simulink subsystem "SerialTX"  (R2022a)
settings: Solver=VariableStepAuto  StartTime=0.0  StopTime=10.0  RelTol=1e-3
undefined symbols (not defined in the file): A0, A1, PTB2, PTB3
libraries: frdmk64flib x3
settings Model: Creator=bkfre  LastModifiedBy=bkfre

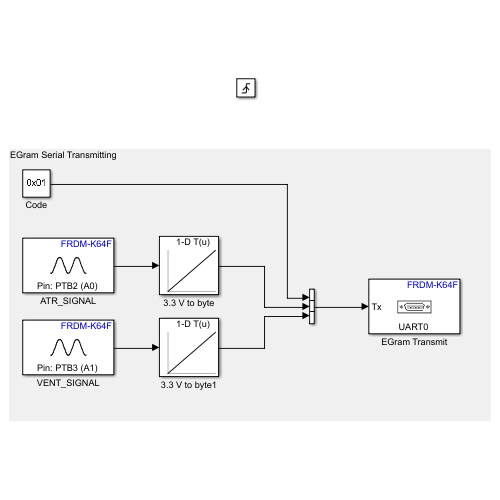
[thumbnail: Simulink's stored preview of the top-level diagram]
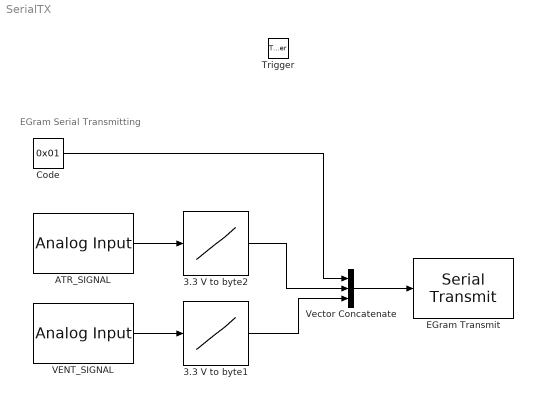
== system SerialTX ==
  note: EGram Serial Transmitting
  Trigger : TriggerPort  VariantControl=(inherit)  PortDimensions=1
  3.3 V to byte1 : Lookup_n-D  NumberOfTableDimensions=1  BreakpointsForDimension1=[0,3.3]  Table=[0,255]  ExtrapMethod=Clip  InternalRulePriority=Speed  OutDataTypeStr=uint8  RndMeth=Simplest
  3.3 V to byte2 : Lookup_n-D  NumberOfTableDimensions=1  BreakpointsForDimension1=[0,3.3]  Table=[0,255]  ExtrapMethod=Clip  InternalRulePriority=Speed  OutDataTypeStr=uint8  RndMeth=Simplest
  ATR_SIGNAL : frdmk64flib/Analog Input  Whichpin=PTB2 (A0)  SampleTime=-1
  Code : Constant  Value=0x01  OutDataTypeStr=uint8
  EGram Transmit : frdmk64flib/Serial Transmit  SCIModule=0  Baudrate=uint32(9600)  Parity=None  StopBits=1  HardwareFlowControl=None  ByteOrder=LittleEndian  BlockingMode=on  OutputStatus=off
  VENT_SIGNAL : frdmk64flib/Analog Input  Whichpin=PTB3 (A1)  SampleTime=-1
  Vector Concatenate : Concatenate  NumInputs=3
  wires:
  ATR_SIGNAL/1 -> 3.3 V to byte2/1
  3.3 V to byte1/1 -> Vector Concatenate/3
  Vector Concatenate/1 -> EGram Transmit/1
  Code/1 -> Vector Concatenate/1
  3.3 V to byte2/1 -> Vector Concatenate/2
  VENT_SIGNAL/1 -> 3.3 V to byte1/1
